simulink model "eksperyment1"  (R2017a)
settings: Solver=VariableStepAuto  StartTime=0.0  StopTime=10.0  MaxStep=0.1  MinStep=0.001  RelTol=1e-5
settings Model: Creator=Szwank  LastModifiedBy=Szwank

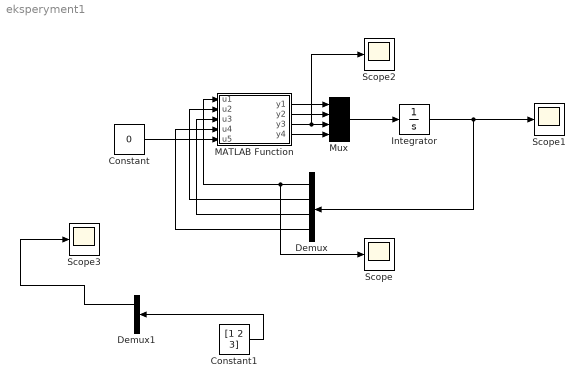
== system eksperyment1 ==
  Constant : Constant  Value=0
  Constant1 : Constant  Value=[1 2 3]
  Demux : Demux
  Demux1 : Demux  Outputs=3
  Integrator : Integrator  InitialCondition=[0 pi 0 0]
  MATLAB Function : MATLAB Function  TreatAsAtomicUnit=on
  Mux : Mux
      settings: DisplayOption=signals
  Scope{,1..3} (4 alike) : Scope
  wires:
  Mux/1 -> Integrator/1
  MATLAB Function/1(y1) -> Mux/1
  MATLAB Function/2(y2) -> Mux/2
  MATLAB Function/3(y3) -> Scope2/1, Mux/3
  MATLAB Function/4(y4) -> Mux/4
  Integrator/1 -> Demux/1, Scope1/1
  Constant/1 -> MATLAB Function/5(u5)
  Constant1/1 -> Demux1/1
  Demux1/1 -> Scope3/1
  Demux/1 -> Scope/1, MATLAB Function/1(u1)
  Demux/2 -> MATLAB Function/2(u2)
  Demux/3 -> MATLAB Function/3(u3)
  Demux/4 -> MATLAB Function/4(u4)

== matlab function eksperyment1/MATLAB Function ==
  data: u1 input; y1 output; u2 input; u3 input; u4 input; u5 input; y2 output; y3 output; y4 output
function [y1,y2,y3,y4] = fcn(u1,u2,u3,u4,u5)
%Dane obiektu
%% Motor
Rm = 3.3; % ohms, Motor armature resistance 
Kt = 0.0280; % N.m, Motor torque constant
Km = 0.0280; % V/(rad/s), Motor back-emf constant (same as Ktin SI units)
Jm = 9.64e-6; % kg.m2, Moment of inertia of motor rotor. 
Jeq = 1.23e-4; % kg.m2, Equivalent moment of inertia about motor shaft pivot axis.
%% Pendulum Arm:
Marm = 0.0280; % kg, Mass of the arm.
r = 0.0826; % m, Length of arm pivot to pendulum pivot.
Beq = 0.1; % N.m/(rad/s), Arm viscous damping. 
%% Pendulum Link:
Mp = 0.0270; % kg, Mass of the pendulum link and weight combined.
Lp = 0.191; % m, Total length of pendulum.
lp = 0.153; % m, Length of pendulum center of mass from pivot.
Jp = 1.20e-4; % kg.m2, Pendulum moment of inertia about its pivot axis.
Bp = 0; % N.m/(rad/s), Pendulum viscous damping.
%% Pulse-Width Modulated Amplifier:
Vmax = 24; % V, PWM amplifier maximum output voltage
PWM = 5; % A, amplifier maximum output current
Kw = 2.3; % V/V, PWM amplifier gain
%% Stałe
m = Mp;
g = 9.80665;
a = Jeq + m * r^2;
b = m * lp * r;
e = m*lp^2 + Jp;
f = m*g*lp;
c = Km*Kw/Rm;
d = (Km*Kt+Beq*Rm)/Rm;
%%

y1 = u3;
y2 = u4;
y3 = 1/(1-(b^2/(a*e))*cos(u2)^2)*(1/a)*(b*f/e*sin(u2)*cos(u2)-b*u4^2*sin(u2)+u5*c-d*u3);
y4 = 1/(1-(b^2/(a*e))*cos(u2)^2)*(1/e)*(b/a*cos(u2)*(-b*u4^2*sin(u2)+c*u5-d*u3)+f*sin(u2));
